simulink model "power_calc"  (R2020a)
settings: Solver=VariableStepAuto  StartTime=0.0  StopTime=10  RelTol=1e-3
model workspace (MAT data in the model file):
  f = 60
libraries: powerlib x5
settings Model: Creator=Krish  LastModifiedBy=Krish
settings OptimizationCC: ZeroExternalMemoryAtStartup=off  ZeroInternalMemoryAtStartup=off
settings RTWCC: GenCodeOnly=on  TargetLang=C++  CheckMdlBeforeBuild=Warning
settings GRTTargetCC: TargetLangStandard=C++03 (ISO)  MultiInstanceERTCode=on  CodeInterfacePackaging=C++ class

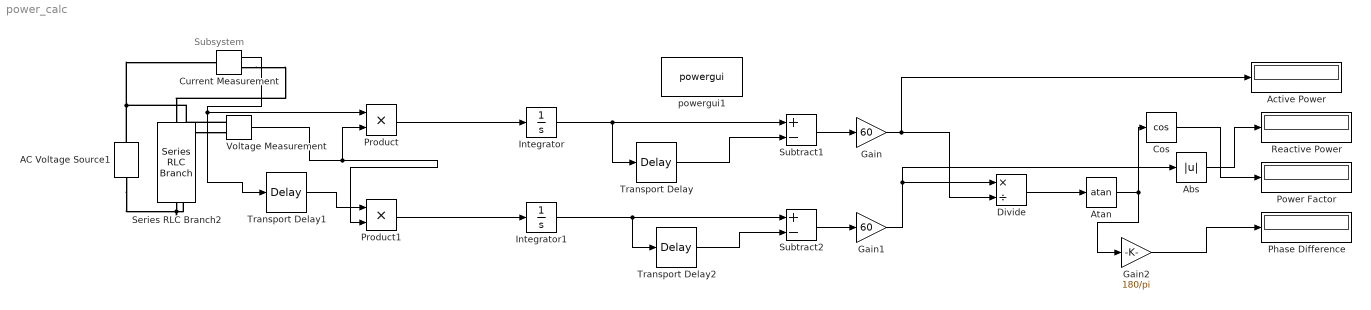
== system power_calc ==
  note: Subsystem
  AC Voltage Source1 : powerlib/Electrical Sources/AC Voltage Source  Amplitude=320  Phase=0  Frequency=60  SampleTime=0  Measurements=None  BusType=swing  Pref=10e3  Qref=0  Qmin=-inf  Qmax=+inf
  Abs : Abs
  Active Power : Display
  Atan : Trigonometry  Operator=atan
  Cos : Trigonometry  Operator=cos
  Current Measurement : powerlib/Measurements/Current Measurement  PhasorSimulation=off  OutputType=Complex  PSBequivalent=0
  Divide : Product  Inputs=*/
  Gain : Gain  Gain=60
  Gain1 : Gain  Gain=60
  Gain2 : Gain  Gain=180/pi
  Integrator : Integrator
  Integrator1 : Integrator
  Phase Difference : Display
  Power Factor : Display
  Product : Product
  Product1 : Product
  Reactive Power : Display
  Series RLC Branch2 : powerlib/Elements/Series RLC Branch  LConnTagsString=__new0  RConnTagsString=__new0  BranchType=RL  Resistance=100  Inductance=1e-1  SetiL0=off  InitialCurrent=0  Capacitance=1e-6  Setx0=off  InitialVoltage=0  Measurements=None
  Subtract1 : Sum  Inputs=+-
  Subtract2 : Sum  Inputs=+-
  Transport Delay : TransportDelay  DelayTime=1/60
  Transport Delay1 : TransportDelay  DelayTime=1/240
  Transport Delay2 : TransportDelay  DelayTime=1/60
  Voltage Measurement : powerlib/Measurements/Voltage Measurement  PhasorSimulation=off  OutputType=Complex  PSBequivalent=0
  powergui1 : powerlib/powergui  Priority=1  SimulationMode=Continuous  SampleTime=50e-6  frequency=60  Iterations=50  frequencyindice=60  Pbase=100e6  ErrMax=1e-4  UnitsV=kV  UnitsW=MW  buscounter=0  FunctionMessages=off  echomessages=off  EnableUseOfTLC=off  CurrentSourceSwitches=off  DisableSnubberDevices=off  DisableRonSwitches=off  DisableVfSwitches=off  DisplayEquations=off  AutomaticDiscreteSolvers=off  SolverType=Tustin/Backward Euler (TBE)  Interpol=off  ExternalGateDelay=off  methode=off  Ts=100  x0status=blocks  SPID=on  SwTol=0  HookPort=off  NonlinearTolerance=1e-4  nMaxIteration=100  ContinueOnMaxIteration=off  RestoreLinks=warning  ResistiveCurrentMeasurement=off  Frange=[0:2:500]  Ylog=off  Xlog=on  ShowGrid=off  save=off  variable=ZData  structure=0  ZoomFFT=off  StartTime=0.0  cycles=1  DisplayStyle=1  fundamental=60  FreqAxis=off  MaxFrequency=1000  frequencyindicesteady=1  RmsSteady=1  display=off
  wires:
  Subtract2/1 -> Gain1/1
  Atan/1 -> Gain2/1, Cos/1
  Divide/1 -> Atan/1
  Integrator1/1 -> Subtract2/1, Transport Delay2/1
  Product1/1 -> Integrator1/1
  Subtract1/1 -> Gain/1
  Transport Delay2/1 -> Subtract2/2
  Integrator/1 -> Subtract1/1, Transport Delay/1
  Gain2/1 -> Phase Difference/1
  Transport Delay1/1 -> Product1/1
  Voltage Measurement/1 -> Product1/2, Product/2
  Gain1/1 -> Divide/1, Abs/1
  Current Measurement/1 -> Transport Delay1/1, Product/1
  Cos/1 -> Power Factor/1
  Product/1 -> Integrator/1
  Transport Delay/1 -> Subtract1/2
  Gain/1 -> Divide/2, Active Power/1
  Abs/1 -> Reactive Power/1
  connections:
  Series RLC Branch2/RConn1 -- AC Voltage Source1/LConn1 -- Voltage Measurement/LConn2
  Voltage Measurement/LConn1 -- Current Measurement/LConn1 -- AC Voltage Source1/RConn1
  Current Measurement/RConn1 -- Series RLC Branch2/LConn1
